simulink model "led_count"  (R2014a)
settings: Solver=ode3  StartTime=0.0  StopTime=1000  FixedStep=1  RelTol=1e-3
libraries: hdlsllib x10, simulink x1
settings Model: Creator=Shiyu  LastModifiedBy=wang.shiyu
settings OptimizationCC: BlockReduction=off  ConditionallyExecuteInputs=off  InlineParams=on
settings DebuggingCC: AlgebraicLoopMsg=error
settings HardwareCC: ProdHWDeviceType=ASIC/FPGA->ASIC/FPGA  ProdEqTarget=off

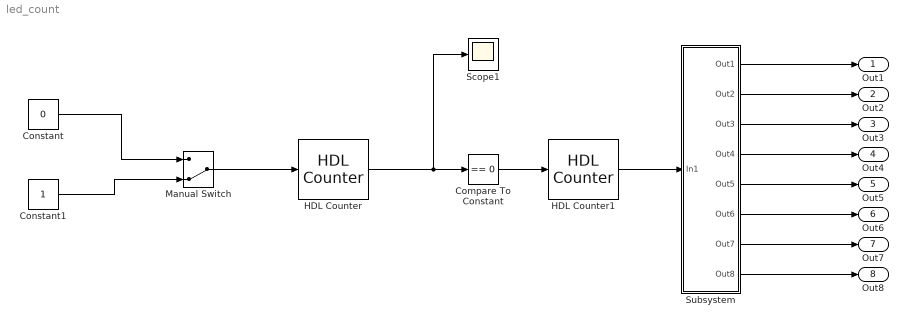
== system led_count ==
  Compare To Constant : simulink/Logic and Bit Operations/Compare To Constant  relop===  const=0  OutDataTypeStr=boolean
  Constant : Constant  Value=0  OutDataTypeStr=boolean
  Constant1 : Constant  OutDataTypeStr=boolean
  HDL Counter : hdlsllib/HDL Operations/HDL Counter  CountType=Count limited  CountInit=0  CountStep=1  CountMax=25  CountFromType=Initial value  CountFrom=0  CountResetPort=off  CountLoadPort=off  CountEnbPort=on  CountDirPort=off  CountDataType=Unsigned  CountWordLen=8  CountFracLen=0  CountSampTime=1
  HDL Counter1 : hdlsllib/HDL Operations/HDL Counter  CountType=Free running  CountInit=0  CountStep=1  CountMax=100  CountFromType=Initial value  CountFrom=0  CountResetPort=off  CountLoadPort=off  CountEnbPort=on  CountDirPort=off  CountDataType=Unsigned  CountWordLen=8  CountFracLen=0  CountSampTime=1
  Manual Switch : ManualSwitch  CurrentSetting=0
  Scope1 : Scope
  Subsystem : Subsystem  TreatAsAtomicUnit=on
  Out1 : Outport
  Out2 : Outport  Port=2
  Out3 : Outport  Port=3
  Out4 : Outport  Port=4
  Out5 : Outport  Port=5
  Out6 : Outport  Port=6
  Out7 : Outport  Port=7
  Out8 : Outport  Port=8
  wires:
  Constant1/1 -> Manual Switch/2
  Constant/1 -> Manual Switch/1
  Manual Switch/1 -> HDL Counter/1
  HDL Counter/1 -> Scope1/1, Compare To Constant/1
  Compare To Constant/1 -> HDL Counter1/1
  HDL Counter1/1 -> Subsystem/1(In1)
  Subsystem/1(Out1) -> Out1/1
  Subsystem/3(Out3) -> Out3/1
  Subsystem/4(Out4) -> Out4/1
  Subsystem/5(Out5) -> Out5/1
  Subsystem/6(Out6) -> Out6/1
  Subsystem/7(Out7) -> Out7/1
  Subsystem/8(Out8) -> Out8/1
  Subsystem/2(Out2) -> Out2/1

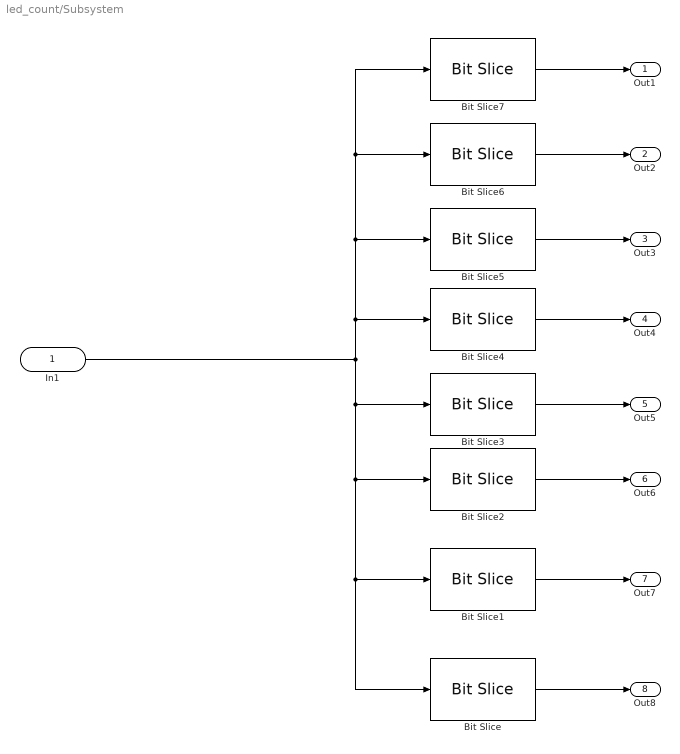
== system led_count/Subsystem ==
  In1 : Inport  OutDataTypeStr=uint8  SampleTime=1  LockScale=on
  Bit Slice : hdlsllib/HDL Operations/Bit Slice  lidx=0  ridx=0
  Bit Slice1 : hdlsllib/HDL Operations/Bit Slice  lidx=1  ridx=1
  Bit Slice2 : hdlsllib/HDL Operations/Bit Slice  lidx=2  ridx=2
  Bit Slice3 : hdlsllib/HDL Operations/Bit Slice  lidx=3  ridx=3
  Bit Slice4 : hdlsllib/HDL Operations/Bit Slice  lidx=4  ridx=4
  Bit Slice5 : hdlsllib/HDL Operations/Bit Slice  lidx=5  ridx=5
  Bit Slice6 : hdlsllib/HDL Operations/Bit Slice  lidx=6  ridx=6
  Bit Slice7 : hdlsllib/HDL Operations/Bit Slice  lidx=7  ridx=7
  Out1 : Outport  SampleTime=1
  Out2 : Outport  Port=2  SampleTime=1
  Out3 : Outport  Port=3  SampleTime=1
  Out4 : Outport  Port=4  SampleTime=1
  Out5 : Outport  Port=5  SampleTime=1
  Out6 : Outport  Port=6  SampleTime=1
  Out7 : Outport  Port=7  SampleTime=1
  Out8 : Outport  Port=8  SampleTime=1
  wires:
  Bit Slice6/1 -> Out2/1
  Bit Slice4/1 -> Out4/1
  Bit Slice5/1 -> Out3/1
  Bit Slice/1 -> Out8/1
  Bit Slice3/1 -> Out5/1
  Bit Slice2/1 -> Out6/1
  Bit Slice1/1 -> Out7/1
  In1/1 -> Bit Slice1/1, Bit Slice/1, Bit Slice2/1, Bit Slice3/1, Bit Slice7/1, Bit Slice6/1, Bit Slice5/1, Bit Slice4/1
  Bit Slice7/1 -> Out1/1
